simulink model "wcusp_circuit"  (Simulink 8.4)
settings: Solver=ode45  StartTime=0.0  StopTime=50  RelTol=1e-6
InitFcn:
  | wcusp_params
values from neighbouring files (symbols this model uses):
  alpha = 0.7    [wcusp_burst_params.m]    (also in wcusp_params.m)
  alpha_peak = 0.3    [wcusp_burst_params.m]    (also in wcusp_params.m)
  beta = 0.5    [wcusp_burst_params.m]    (also in wcusp_params.m)
  delta = 1    [wcusp_burst_params.m]    (also in wcusp_params.m)
  gamma = 0.3    [wcusp_burst_params.m]    (also in wcusp_params.m)
  tau_f = 0.0075    [wcusp_burst_params.m]    (also in wcusp_params.m)
  tau_s = 1    [wcusp_burst_params.m]    (also in wcusp_params.m)
  xf_0 = -1    [wcusp_burst_params.m]    (also in wcusp_params.m)
  xs_0 = -1    [wcusp_burst_params.m]    (also in wcusp_params.m)
libraries: simulink x1
settings Model: Creator=tbb29  LastModifiedBy=tbb29
settings DataIOCC: SignalLoggingSaveFormat=Dataset
settings OptimizationCC: ExpressionDepthLimit=128
settings DebuggingCC: UnderspecifiedInitializationDetection=Simplified  MergeDetectMultiDrivingBlocksExec=error  FcnCallInpInsideContextMsg=EnableAllAsWarning  StateNameClashWarn=none
settings GRTTargetCC: CombineOutputUpdateFcns=on  GRTInterface=off

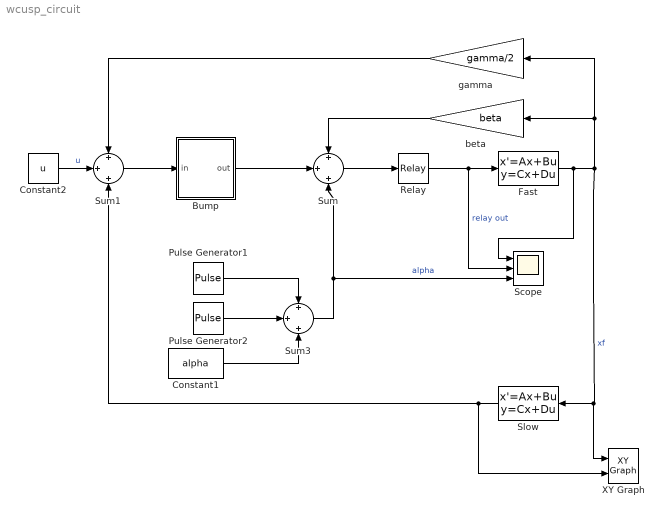
== system wcusp_circuit ==
  Bump : Subsystem
  Constant1 : Constant  Value=alpha
  Constant2 : Constant  Value=u
  Fast : StateSpace  A=-1/tau_f  B=1/tau_f  D=0  X0=xf_0
  Pulse Generator1 : DiscretePulseGenerator  PulseType=Time based  Amplitude=alpha_peak  Period=100  PulseWidth=2  PhaseDelay=10
  Pulse Generator2 : DiscretePulseGenerator  PulseType=Time based  Amplitude=-alpha_peak  Period=100  PulseWidth=2  PhaseDelay=35
  Relay : Relay  OnSwitchValue=0  OffSwitchValue=0  OffOutputValue=-1
  Scope : Scope  NumInputPorts=3
      settings: TimeRange=50  YMin=-1.5~-1~0.4  YMax=1.5~1~0.7
  Slow : StateSpace  A=-1/tau_s  B=1/tau_s  D=0  X0=xs_0
  Sum : Sum  Inputs=+|+|+
  Sum1 : Sum  Inputs=+|+|+
  Sum3 : Sum  Inputs=+|+|+
  XY Graph : simulink/Sinks/XY Graph  xmin=-1  xmax=1  ymin=-1  ymax=1  st=-1
  beta : Gain  Gain=beta
  gamma : Gain  Gain=gamma/2
  wires:
  Sum/1 -> Relay/1
  beta/1 -> Sum/1
  Relay/1 -> Fast/1, Scope/2  "relay out"
  Fast/1 -> beta/1, gamma/1, Slow/1, XY Graph/1, Scope/1  "xf"
  Bump/1(out) -> Sum/2
  Slow/1 -> Sum1/3, XY Graph/2
  Pulse Generator2/1 -> Sum3/2
  Pulse Generator1/1 -> Sum3/1
  Constant1/1 -> Sum3/3
  Constant2/1 -> Sum1/2  "u"
  gamma/1 -> Sum1/1
  Sum3/1 -> Sum/3, Scope/3  "alpha"
  Sum1/1 -> Bump/1(in)

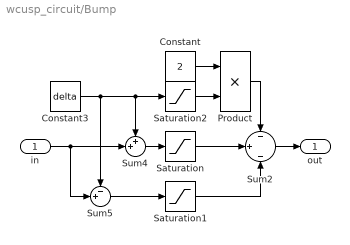
== system wcusp_circuit/Bump ==
  in : Inport
  Constant : Constant  Value=2
  Constant3 : Constant  Value=delta
  Product : Product  RndMeth=Zero
  Saturation : Saturate  UpperLimit=1  LowerLimit=-1
  Saturation1 : Saturate  UpperLimit=1  LowerLimit=-1
  Saturation2 : Saturate  UpperLimit=1  LowerLimit=-1
  Sum2 : Sum  Inputs=-|+|-
  Sum4 : Sum  Inputs=++|
  Sum5 : Sum  Inputs=-+|
  out : Outport
  wires:
  Saturation1/1 -> Sum2/3
  Saturation/1 -> Sum2/2
  Product/1 -> Sum2/1
  Saturation2/1 -> Product/2
  Constant/1 -> Product/1
  Constant3/1 -> Saturation2/1, Sum4/1, Sum5/1
  Sum4/1 -> Saturation/1
  in/1 -> Sum5/2, Sum4/2
  Sum5/1 -> Saturation1/1
  Sum2/1 -> out/1
